simulink model "SimpleStateMachine"  (Simulink 8.0)
settings: Solver=FixedStepDiscrete  StartTime=0.0  StopTime=2*pi  FixedStep=.05  RelTol=1e-3
settings Model: Creator=LukePH  LastModifiedBy=Luke
settings OptimizationCC: ExpressionDepthLimit=128
settings DebuggingCC: StateNameClashWarn=none
settings CodeAppCC: CustomSymbolStrType=$N$R$M_T  InternalIdentifier=Shortened

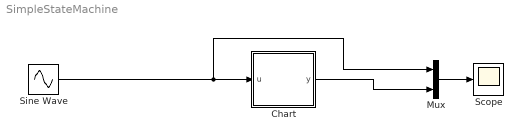
== system SimpleStateMachine ==
  Chart : Stateflow chart  TreatAsAtomicUnit=on
  Mux : Mux  Inputs=2
  Scope : Scope
  Sine Wave : Sin  SampleTime=0
  wires:
  Sine Wave/1 -> Mux/1, Chart/1(u)
  Chart/1(y) -> Mux/2
  Mux/1 -> Scope/1

== stateflow chart Chart ==
  state On
    entry: y = 1;
  state OFF
    entry: y = -1;
  (default) -> On
  On -> OFF : [u<0]
  OFF -> On : [u>0]
  data: u input double; y output double
